simulink model "arrayProcessingBlock"  (R2012b)
settings: Solver=FixedStepDiscrete  StartTime=0.0  StopTime=10.0  FixedStep=0.001  RelTol=1e-3
settings Model: BufferReuse=off  Creator=gilja  LastModifiedBy=Chethan
settings SolverCC: EnableConcurrentExecution=on  ConcurrentTasks=on
settings DataIOCC: SaveOutput=off  SignalLogging=off  DSMLogging=off  SaveTime=off
settings OptimizationCC: InlineParams=on  InlineInvariantSignals=on  OptimizeBlockIOStorage=off  BufferReuse=off  ExpressionFolding=off  LocalBlockOutputs=off
settings HardwareCC: ProdIntDivRoundTo=Zero  ProdEndianess=LittleEndian  ProdHWDeviceType=Generic->32-bit x86 compatible
settings ModelReferenceCC: ModelReferenceMinAlgLoopOccurrences=on
settings RTWCC: SystemTargetFile=xpctarget.tlc  TemplateMakefile=xpc_default_tmf  Description=xPC Target  ProcessScript=xpctarget_make_rtw_hook  RTWCompilerOptimization=On
settings CodeAppCC: MaxIdLength=62
settings xpcTargetCC: TargetFcnLib=ansi_tfl_table_tmw.mat  CodeReplacementLibrary=XPC_BLAS  ParMdlRefBuildCompliant=on  ConcurrentExecutionCompliant=on  CombineSignalStateStructs=off  GRTInterface=on  xPCTaskExecutionProfile=on  xPCRL32EventNumber=5000  xPCisDownloadable=off  xPCLoadParamSetFile=off  xPCConcurrentTasks=off  xPCEnableSFAnimation=off

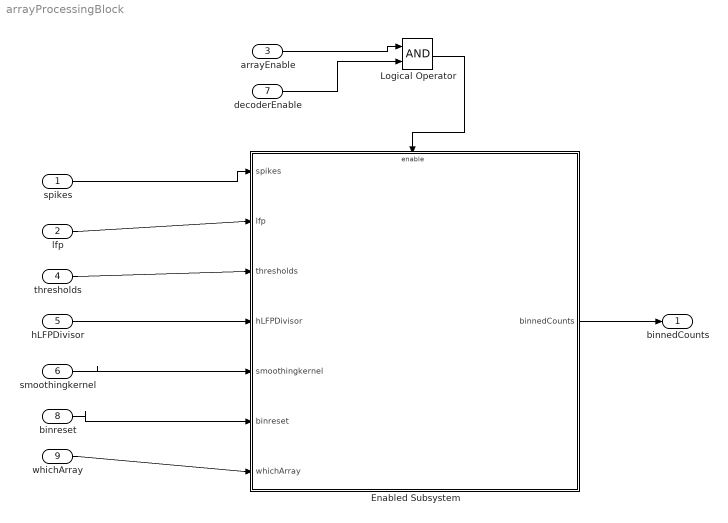
== system arrayProcessingBlock ==
  spikes : Inport  OutDataTypeStr=Bus: processedNeural
  lfp : Inport  Port=2
  arrayEnable : Inport  Port=3  OutDataTypeStr=uint8
  thresholds : Inport  Port=4
  hLFPDivisor : Inport  Port=5
  smoothingkernel : Inport  Port=6
  decoderEnable : Inport  Port=7  OutDataTypeStr=boolean
  binreset : Inport  Port=8
  whichArray : Inport  Port=9
  Enabled Subsystem : Subsystem  TreatAsAtomicUnit=on
  Logical Operator : Logic  AllPortsSameDT=off  OutDataTypeStr=boolean
  binnedCounts : Outport  BusOutputAsStruct=on
  wires:
  spikes/1 -> Enabled Subsystem/1(spikes)
  lfp/1 -> Enabled Subsystem/2(lfp)
  thresholds/1 -> Enabled Subsystem/3(thresholds)
  hLFPDivisor/1 -> Enabled Subsystem/4(hLFPDivisor)
  smoothingkernel/1 -> Enabled Subsystem/5(smoothingkernel)
  binreset/1 -> Enabled Subsystem/6(binreset)
  Logical Operator/1 -> Enabled Subsystem/Enable
  Enabled Subsystem/1(binnedCounts) -> binnedCounts/1
  whichArray/1 -> Enabled Subsystem/7(whichArray)
  decoderEnable/1 -> Logical Operator/2
  arrayEnable/1 -> Logical Operator/1

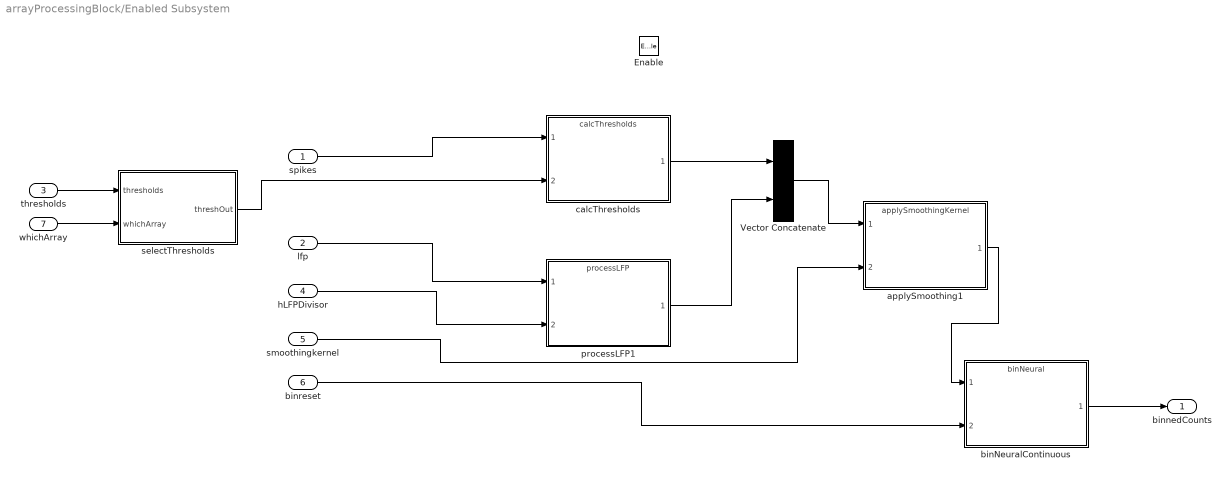
== system arrayProcessingBlock/Enabled Subsystem ==
  spikes : Inport  OutDataTypeStr=Bus: processedNeural
  lfp : Inport  Port=2
  thresholds : Inport  Port=3
  hLFPDivisor : Inport  Port=4
  smoothingkernel : Inport  Port=5
  binreset : Inport  Port=6
  whichArray : Inport  Port=7
  Enable : EnablePort
  Vector Concatenate : Concatenate  Mode=Multidimensional array  ConcatenateDimension=2
  applySmoothing1 : ModelReference  ModelNameDialog=applySmoothingKernel  SimulationMode=Normal  ModelReferenceVersion=1.46  CopyOfModelName=applySmoothingKernel  DefaultDataLogging=on
  binNeuralContinuous : ModelReference  ModelNameDialog=binNeural  SimulationMode=Normal  ModelReferenceVersion=1.47  CopyOfModelName=binNeural  DefaultDataLogging=on
  calcThresholds : ModelReference  ModelNameDialog=calcThresholds  SimulationMode=Normal  ModelReferenceVersion=1.50  CopyOfModelName=calcThresholds  DefaultDataLogging=on
  processLFP1 : ModelReference  ModelNameDialog=processLFP  SimulationMode=Normal  ModelReferenceVersion=1.60  CopyOfModelName=processLFP  DefaultDataLogging=on
  selectThresholds : MATLAB Function  TreatAsAtomicUnit=on
  binnedCounts : Outport  BusOutputAsStruct=on
  wires:
  calcThresholds/1 -> Vector Concatenate/1
  processLFP1/1 -> Vector Concatenate/2
  lfp/1 -> processLFP1/1
  spikes/1 -> calcThresholds/1
  applySmoothing1/1 -> binNeuralContinuous/1
  Vector Concatenate/1 -> applySmoothing1/1
  hLFPDivisor/1 -> processLFP1/2
  smoothingkernel/1 -> applySmoothing1/2
  binreset/1 -> binNeuralContinuous/2
  binNeuralContinuous/1 -> binnedCounts/1
  whichArray/1 -> selectThresholds/2(whichArray)
  thresholds/1 -> selectThresholds/1(thresholds)
  selectThresholds/1(threshOut) -> calcThresholds/2

== matlab function arrayProcessingBlock/Enabled Subsystem/selectThresholds ==
  data: thresholds input size=[192 1]; whichArray input double; threshOut output size=[96 1]
function threshOut = selectNeuralChannels(thresholds, whichArray)
%#codegen
persistent threshOutTmp
if(isempty(threshOutTmp))
    threshOutTmp = zeros([96 1])+200;
end

threshOutTmp(:,1) = thresholds((1:96)+96*(whichArray-1),1);

threshOut = threshOutTmp;
